simulink model "CM650A_HwTq0Meas"  (R2013b)
settings: Solver=FixedStepDiscrete  StartTime=0.0  StopTime=20  FixedStep=0.002  RelTol=1e-3
values from neighbouring files (symbols this model uses):
  ELECGLBPRM_HWTQOFFS_HWNWTMTR_F32 = DataDict.Constant    [CM650A_HwTq0Meas_DataDict.m]
  ELECGLBPRM_HWTQSATNLOWRLIM_HWNWTMTR_F32 = DataDict.Constant    [CM650A_HwTq0Meas_DataDict.m]
  ELECGLBPRM_HWTQSATNUPPRLIM_HWNWTMTR_F32 = DataDict.Constant    [CM650A_HwTq0Meas_DataDict.m]
  ELECGLBPRM_HWTQSCA_ULS_F32 = DataDict.Constant    [CM650A_HwTq0Meas_DataDict.m]
  ELECGLBPRM_NOFLT_CNT_U08 = DataDict.Constant    [CM650A_HwTq0Meas_DataDict.m]
  ELECGLBPRM_OFFSTRIMNOTPRFM_CNT_U08 = DataDict.Constant    [CM650A_HwTq0Meas_DataDict.m]
  ELECGLBPRM_PRTCLFLT_CNT_U08 = DataDict.Constant    [CM650A_HwTq0Meas_DataDict.m]
  ELECGLBPRM_SNSRINTFLT_CNT_U08 = DataDict.Constant    [CM650A_HwTq0Meas_DataDict.m]
  FLTINJ_HWTQ0MEAS_HWTQ0 = DataDict.Constant    [CM650A_HwTq0Meas_DataDict.m]
  FLTINJ_HWTQ0MEAS_TESTOK0 = DataDict.Constant    [CM650A_HwTq0Meas_DataDict.m]
  HwTq0MeasHwTq0PrtclFltFailStep = DataDict.Calibration    [CM650A_HwTq0Meas_DataDict.m]
  HwTq0MeasHwTq0PrtclFltPassStep = DataDict.Calibration    [CM650A_HwTq0Meas_DataDict.m]
  RACKLIMRCCWEOTSCA_ULS_F32 = DataDict.Constant    [CM650A_HwTq0Meas_DataDict.m]
  RACKLIMRCWEOTSCA_ULS_F32 = DataDict.Constant    [CM650A_HwTq0Meas_DataDict.m]
undefined symbols (not defined in the file or in its folder): NtcNr1, NtcSts1, sigbuilder_block, SigQlfr1
libraries: simulink x23, NxtrNvM x3, NxtrLim x2
(part 1 of 3)
settings Model: CovMetricSettings=dcmtrzoiw  CovFilter=CM650A_HwTq0Meas_covfilter  CovHTMLOptions=-sRT=1 -aTS=1 -bRG=1 -bTC=1 -hTR=0 -nFC=0 -scm=1 -bcm=1 -xEv=0  CovModelRefEnable=off  BufferReuse=off  Creator=CZ68DS  LastModifiedBy=FZG88Y
settings SolverCC: AutoInsertRateTranBlk=on
settings DataIOCC: SaveFormat=StructureWithTime
settings OptimizationCC: BlockReduction=off  DefaultUnderspecifiedDataType=single  OptimizeBlockIOStorage=off  BufferReuse=off  ExpressionFolding=off  LocalBlockOutputs=off  OptimizeModelRefInitCode=on  LifeSpan=1
settings DebuggingCC: MultiTaskDSMMsg=warning  FrameProcessingCompatibilityMsg=error
settings HardwareCC: ProdIntDivRoundTo=Zero  ProdEndianess=LittleEndian  ProdHWDeviceType=Generic->Custom  TargetIntDivRoundTo=Zero  TargetEndianess=LittleEndian  TargetHWDeviceType=Generic->Custom
settings RTWCC: SystemTargetFile=ert.tlc  TemplateMakefile=ert_default_tmf  Description=Embedded Coder  ProcessScript=ert_make_rtw_hook
settings CodeAppCC: IgnoreCustomStorageClasses=off
settings ERTTargetCC: CodeReplacementLibrary=C89/C90 (ANSI)  GenerateSampleERTMain=on  ERTCustomFileTemplate=example_file_process.tlc

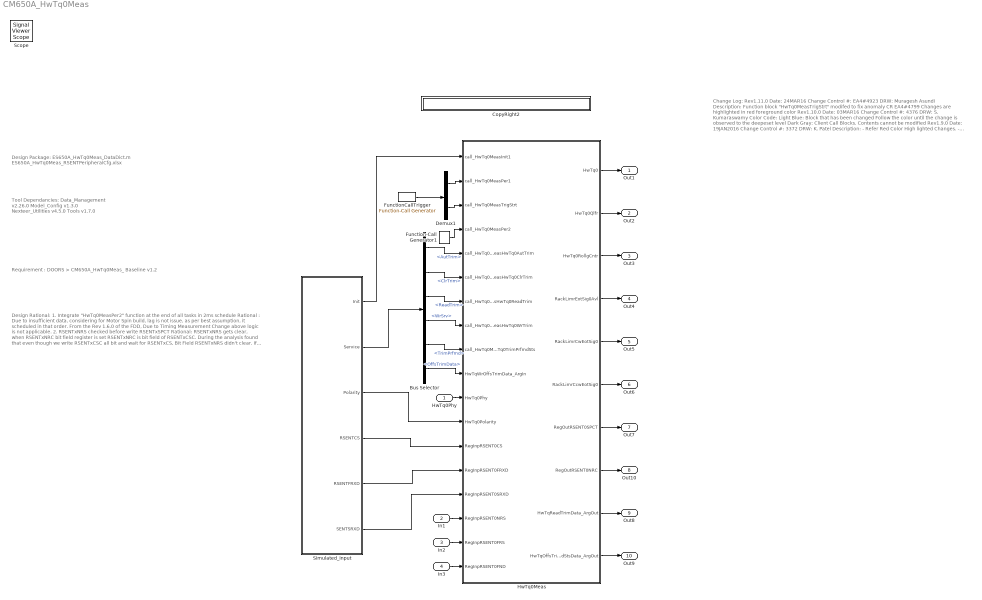
== system CM650A_HwTq0Meas ==
  note: Design Package:
      |
      | ES650A_HwTq0Meas_DataDict.m
      | ES650A_HwTq0Meas_RSENTPeripheralCfg.xlsx
  note: Change Log:
      |
      | Rev1.11.0
      | Date: 24MAR16
      | Change Control #: EA4#4923
      | DRW: Muragesh Asundi
      | Description:
      | Function block "HwTq0MeasTrigStrt" modifed to fix anomaly CR EA4#4799
      | Changes are highlighted in red foreground color
      |
      | Rev1.10.0
      | Date: 03MAR16
      | Change Control #: 4376
      | DRW: S. Kumaraswamy
      | Color Code:
      | Light Blue:	Block that has been changed
      | 				Follow the color until the change is observed to the deepeset level
      | Dark Gray:	Client Call Blocks. Contents cannot be modified
      |
      | Rev1.9.0
      | Date: 19JAN2016
      | Change Control #: 3372
      | DRW: K. Patel
      | Description:
      | - Refer Red Color High lighted Changes.
      | -  "CM650A_HwTq0Meas_RSENTPeripheralCfg.xlsx" change
      |
      | Rev1.8.0
      | Date: 16DEC2015
      | Change Control #: 3155
      | DRW: K. Patel
      | Description:
      | - Refer Red Color High lighted Changes.
      |
      | Rev1.7.0
      | Date: 22OCT2015
      | Change Control #: EA4#2221
      | DRW: K. Patel
      | Description:
      | - Slow Serial Message Fix
      | - EA4 Naming Correction for HwTq0MeasTrigStart
      |
      | Rev1.6.0
      | Date: 09OCT2015
      | Change Control #: EA4#1919
      | DRW: K. Patel
      | Description:
      | - Torque Trigger server function, Per3 change to Per2, Missing Message Counter add per1,
      | remove register from "CM650A_HwTq0Meas_RSENTPeripheralCfg.xlsx", change sync time to 16
      |
      | Rev1.5.0
      | Date: 02OCT2015
      | Change Control #: EA4#1811
      | DRW: Pallav G/Muragesh A (KPIT)
      | Description:
      | - Corrected output signal names RickLimrCcwEotSig0, RickLimrCwEotSig0 to RackLimrCcwEotSig0 and RackLimrCwEotSig0 respectively
      | - Range limiter added for above two output signals
      |
      | Rev1.4.0
      | Date: 20AUG2015
      | Change Control #: WCR-EA4#1283
      | DRW: K. Patel
      | Description:
      | - Rack Limiter End of Travel Signal 0 Data Read Function added
      |
      | Rev1.3.0
      | Date: 30JUL2015
      | Change Control #: WCR-EA4#1163, EA4#1222
      | DRW: K. Patel
      | Description:
      | - m file correction, Tick Time change from 1us to 1.2us
      | - Global Constant
      |
      | Rev1.2.0
      | Date: 29JUN2015
      | Change Control #: WCR-EA4#993
      | DRW: K. Patel
      | Description:
      | - Fault Injection added
      | - Trim Services Added
      | - Remove Mask in protocol evaluation & use field level register for input
      |
      | Rev1.1.0
      | Date: 30MAR2015
      | Change Control #: WCR-EA4#531
      | DRW: K. Patel
      | Description:
      | - Constant Added to m file and name corrected as per autosar
      | - Configuration Change in Init added
      |
      | Rev: 1.0.1
      | Date: 30MAR2015
      | Change Control #: WCR-EA4#425
      | DRW: K. Patel
      | Description:
      | - DebStep Cal range change and unit corrected in M file
      | - HwTq0Phy terminate out side of Init function as per Software Recommandation
      | - HwTq0MeasInit start with index 1 corrected as per EA4 meeting decision
      |
      | DRW: Keyur Patel
      | Description:
      | - Model intent to implement EA4 SENT0 based Digital Torque implementation for T1xx.
      |    model runs at three different function rate:
      |       1) Init - Configure Peripheral
      |       2) 2ms - Running SENT data, protocol fault, HwNm calculation, SENT trigger.
      |       3) 100ms - Per3 Trim Not Performed evaluation
      |       4) Event Trim Service - Auto, Clear, Write, Read, Trim Performed Status
      | - Fault Injection added
      | - Copyright Blocks added to each layer
      |
      | Rev: 100
      | Date: 6MAR2015
      | Change Control #: WCR-EA4#152
      | DRW: K. Patel
      | Description:
      | - Initial Release
  note: Tool Dependancies:
      |
      | Data_Management v2.26.0
      | Model_Config v1.3.0
      | Nexteer_Utilities v4.5.0
      | Tools v1.7.0
  note: Requirement :
      |
      | DOORS > CM650A_HwTq0Meas_ Baseline v1.2
  note: Design Rational:
      |
      | 1. Integrate "HwTq0MeasPer2" function at the end of all tasks in 2ms schedule
      | Rational : Due to insufficient data, considering for Motor Spin build, lag is not
      | issue, as per best assumption, it scheduled in that order.
      |
      | From the Rev 1.6.0 of the FDD, Due to Timing Measurement Change above
      | logic is not applicable.
      |
      | 2. RSENTxNRS checked before write RSENTxSPCT
      | Rational: RSENTxNRS gets clear, when RSENTxNRC bit field register is set
      | RSENTxNRC is bit field of RSENTxCSC. During the analysis found that
      | even though we write RSENTxCSC all bit and wait for RSENTxCS, Bit Field
      | RSENTxNRS didn't clear. If RSENTxNRS is set then writing RSENTxSPCT,
      | Peripheral will not output Pulse.
      |
      | Also found that RSENTxCS didn't clear itself, so need to always clear after
      | read message.
      |
      | 3. RSENTxSPCT need to write first to verify RSENTxNRS status
      | Rational : As per the Renesas User's hardware manual v1.0 -
      | Section 19 -SPC function, "Writing to RSENTnSPCT.TLL requests a
      | SPC trigger transmission. After writing to RSENTnSPCT.TLL, the CPU
      | should read RSENTnCS.NRS to check whether the previous request was
      | completed or not."
  HwTq0Phy : Inport
  In1 : Inport  Port=2
  In2 : Inport  Port=3
  In3 : Inport  Port=4
  Bus Selector : BusSelector  OutputSignals=AutTrim,ClrTrim,ReadTrim,WrSrv,TrimPrfmd,OffsTrimData
  CopyRight2 : Subsystem  Description=|  mask(Copyright Information){none=on}
      | Copyright info block.                                               
      |                                                                     
      | Place copyright information at the top of every subsystem in design.
      mask prompts: none "No parameters"
      mask help: Place copyright information at the top of every subsystem in design.
      mask Display:
      | NxtrConf = 'Nexteer Confidential';
      | 
      | sys = bdroot; %handle for the current model ("system")
      | first = get_param(sys,'Created');
      | first = first(end-3:end);  %year is last four digits
      | 
      | last = get_param(sys,'LastModifiedDate');
      | if isempty(last)
      |     last = datestr(now,'yyyy');
      | else
      |     last = last(end-3:end);
      | end
      | 
      | if strcmp(first,last)
      |     fprintf('%s -- Copyright %s Nexteer',NxtrConf,first)
      | else
      |     fprintf('%s -- %s%s- %s Nexteer',NxtrConf,char(169),first,last)
      | end
  Demux1 : Demux  Outputs=2
  Function-Call Generator1 : simulink/Ports & Subsystems/Function-Call Generator  sample_time=0.100  numberOfIterations=1
  FunctionCallTrigger : simulink/Ports & Subsystems/Function-Call Generator  RequirementInfo={} %GIDa_461051ca_e299_4da2_91c0_e73e41056377  sample_time=0.002  numberOfIterations=1
  HwTq0Meas : Subsystem  Priority=1
      settings: AttributesFormatString=Priority = %<Priority>
  Simulated_Input : Subsystem  Description=Do not Code this block
      settings: AttributesFormatString=%<Description>
  Out1 : Outport
  Out2 : Outport  Port=2
  Out3 : Outport  Port=3
  Out4 : Outport  Port=4
  Out5 : Outport  Port=5
  Out6 : Outport  Port=6
  Out7 : Outport  Port=7
  Out10 : Outport  Port=8
  Out8 : Outport  Port=9
  Out9 : Outport  Port=10
  Scope : SignalViewerScope  IOType=viewer  SampleTime=-1  RefreshTime=0.035000
      settings: YMin=-10  YMax=10
  wires:
  FunctionCallTrigger/1 -> Demux1/1
  HwTq0Phy/1 -> HwTq0Meas/11(HwTq0Phy)
  Simulated_Input/3(Polarity) -> HwTq0Meas/12(HwTq0Polarity)
  HwTq0Meas/3(HwTq0RollgCntr) -> Out3/1
  HwTq0Meas/1(HwTq0) -> Out1/1
  HwTq0Meas/2(HwTq0Qlfr) -> Out2/1
  HwTq0Meas/7(RegOutRSENT0SPCT) -> Out7/1
  Function-Call Generator1/1 -> HwTq0Meas/4(call_HwTq0MeasPer2)
  Demux1/1 -> HwTq0Meas/2(call_HwTq0MeasPer1)
  Demux1/2 -> HwTq0Meas/3(call_HwTq0MeasTrigStrt)
  Bus Selector/1 -> HwTq0Meas/5(call_HwTq0MeasHwTq0AutTrim)  "<AutTrim>"
  Bus Selector/2 -> HwTq0Meas/6(call_HwTq0MeasHwTq0ClrTrim)  "<ClrTrim>"
  Bus Selector/3 -> HwTq0Meas/7(call_HwTq0MeasHwTq0ReadTrim)  "<ReadTrim>"
  Bus Selector/4 -> HwTq0Meas/8(call_HwTq0MeasHwTq0WrTrim)  "<WrSrv>"
  Bus Selector/5 -> HwTq0Meas/9(call_HwTq0MeasHwTq0TrimPrfmdSts)  "<TrimPrfmd>"
  Bus Selector/6 -> HwTq0Meas/10(HwTqWrOffsTrimData_ArgIn)  "<OffsTrimData>"
  Simulated_Input/1(Init) -> HwTq0Meas/1(call_HwTq0MeasInit1)
  Simulated_Input/2(Service) -> Bus Selector/1
  Simulated_Input/4(RSENTCS) -> HwTq0Meas/13(RegInpRSENT0CS)
  Simulated_Input/5(RSENTFRXD) -> HwTq0Meas/14(RegInpRSENT0FRXD)
  HwTq0Meas/9(HwTqReadTrimData_ArgOut) -> Out8/1
  HwTq0Meas/10(HwTqOffsTrimPrfmdStsData_ArgOut) -> Out9/1
  HwTq0Meas/4(RackLimrEotSig0Avl) -> Out4/1
  HwTq0Meas/5(RackLimrCwEotSig0) -> Out5/1
  HwTq0Meas/6(RackLimrCcwEotSig0) -> Out6/1
  Simulated_Input/6(SENTSRXD) -> HwTq0Meas/15(RegInpRSENT0SRXD)
  HwTq0Meas/8(RegOutRSENT0NRC) -> Out10/1
  In1/1 -> HwTq0Meas/16(RegInpRSENT0NRS)
  In2/1 -> HwTq0Meas/17(RegInpRSENT0FRS)
  In3/1 -> HwTq0Meas/18(RegInpRSENT0FND)

== system CM650A_HwTq0Meas/CopyRight2 ==

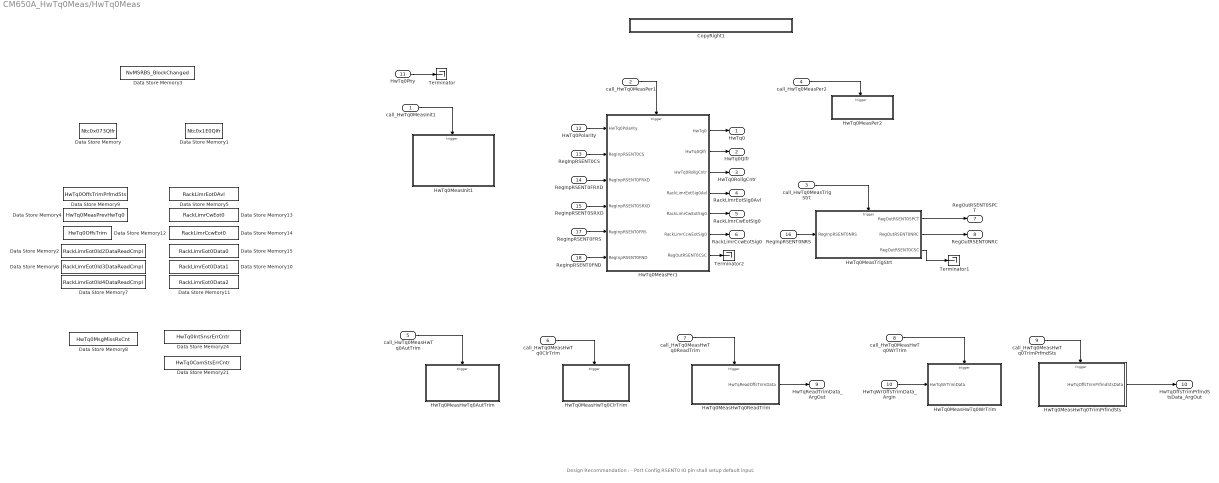
== system CM650A_HwTq0Meas/HwTq0Meas ==
  note: Design Recommandation :
      |
      | - Port Config RSENT0 IO pin shall setup default input.
  call_HwTq0MeasInit1 : Inport
  call_HwTq0MeasPer1 : Inport  Description=2ms  Port=2
      settings: AttributesFormatString=%<Description>
  call_HwTq0MeasTrigStrt : Inport  Description=Event  Port=3
      settings: AttributesFormatString=%<Description>
  call_HwTq0MeasPer2 : Inport  Description=100ms  Port=4
      settings: AttributesFormatString=%<Description>
  call_HwTq0MeasHwTq0AutTrim : Inport  Description=Event  Port=5
      settings: AttributesFormatString=%<Description>
  call_HwTq0MeasHwTq0ClrTrim : Inport  Description=Event  Port=6
      settings: AttributesFormatString=%<Description>
  call_HwTq0MeasHwTq0ReadTrim : Inport  Description=Event  Port=7
      settings: AttributesFormatString=%<Description>
  call_HwTq0MeasHwTq0WrTrim : Inport  Description=Event  Port=8
      settings: AttributesFormatString=%<Description>
  call_HwTq0MeasHwTq0TrimPrfmdSts : Inport  Description=Event  Port=9
      settings: AttributesFormatString=%<Description>
  HwTqWrOffsTrimData_ArgIn : Inport  Port=10
  HwTq0Phy : Inport  Port=11
  HwTq0Polarity : Inport  Port=12  OutDataTypeStr=int8
  RegInpRSENT0CS : Inport  Port=13
  RegInpRSENT0FRXD : Inport  Port=14
  RegInpRSENT0SRXD : Inport  Port=15
  RegInpRSENT0NRS : Inport  Port=16
  RegInpRSENT0FRS : Inport  Port=17
  RegInpRSENT0FND : Inport  Port=18
  CopyRight1 : Subsystem  Description=|  mask(Copyright Information){none=on}
      | Copyright info block.                                               
      |                                                                     
      | Place copyright information at the top of every subsystem in design.
      mask prompts: none "No parameters"
      mask help: Place copyright information at the top of every subsystem in design.
      mask Display:
      | NxtrConf = 'Nexteer Confidential';
      | 
      | sys = bdroot; %handle for the current model ("system")
      | first = get_param(sys,'Created');
      | first = first(end-3:end);  %year is last four digits
      | 
      | last = get_param(sys,'LastModifiedDate');
      | if isempty(last)
      |     last = datestr(now,'yyyy');
      | else
      |     last = last(end-3:end);
      | end
      | 
      | if strcmp(first,last)
      |     fprintf('%s -- Copyright %s Nexteer',NxtrConf,first)
      | else
      |     fprintf('%s -- %s%s- %s Nexteer',NxtrConf,char(169),first,last)
      | end
  Data Store Memory10 : DataStoreMemory  DataStoreName=RackLimrEot0Data1  ReadBeforeWriteMsg=warning  WriteAfterWriteMsg=warning  WriteAfterReadMsg=warning  StateMustResolveToSignalObject=on
  Data Store Memory11 : DataStoreMemory  DataStoreName=RackLimrEot0Data2  ReadBeforeWriteMsg=warning  WriteAfterWriteMsg=warning  WriteAfterReadMsg=warning  StateMustResolveToSignalObject=on
  Data Store Memory12 : DataStoreMemory  DataStoreName=HwTq0OffsTrim  ReadBeforeWriteMsg=warning  WriteAfterWriteMsg=warning  WriteAfterReadMsg=warning
  Data Store Memory13 : DataStoreMemory  DataStoreName=RackLimrCwEot0  ReadBeforeWriteMsg=warning  WriteAfterWriteMsg=warning  WriteAfterReadMsg=warning  StateMustResolveToSignalObject=on
  Data Store Memory14 : DataStoreMemory  DataStoreName=RackLimrCcwEot0  ReadBeforeWriteMsg=warning  WriteAfterWriteMsg=warning  WriteAfterReadMsg=warning  StateMustResolveToSignalObject=on
  Data Store Memory15 : DataStoreMemory  DataStoreName=RackLimrEot0Data0  ReadBeforeWriteMsg=warning  WriteAfterWriteMsg=warning  WriteAfterReadMsg=warning  StateMustResolveToSignalObject=on
  Data Store Memory2 : DataStoreMemory  DataStoreName=RackLimrEot0Id2DataReadCmpl  ReadBeforeWriteMsg=warning  WriteAfterWriteMsg=warning  WriteAfterReadMsg=warning  StateMustResolveToSignalObject=on
  Data Store Memory21 : DataStoreMemory  DataStoreName=HwTq0ComStsErrCntr  ReadBeforeWriteMsg=warning  WriteAfterWriteMsg=warning  WriteAfterReadMsg=warning  StateMustResolveToSignalObject=on
  Data Store Memory24 : DataStoreMemory  DataStoreName=HwTq0IntSnsrErrCntr  ReadBeforeWriteMsg=warning  WriteAfterWriteMsg=warning  WriteAfterReadMsg=warning  StateMustResolveToSignalObject=on
  Data Store Memory4 : DataStoreMemory  DataStoreName=HwTq0MeasPrevHwTq0  ReadBeforeWriteMsg=warning  WriteAfterWriteMsg=warning  WriteAfterReadMsg=warning
  Data Store Memory5 : DataStoreMemory  DataStoreName=RackLimrEot0Avl  ReadBeforeWriteMsg=warning  WriteAfterWriteMsg=warning  WriteAfterReadMsg=warning  StateMustResolveToSignalObject=on
  Data Store Memory6 : DataStoreMemory  DataStoreName=RackLimrEot0Id3DataReadCmpl  ReadBeforeWriteMsg=warning  WriteAfterWriteMsg=warning  WriteAfterReadMsg=warning  StateMustResolveToSignalObject=on
  Data Store Memory7 : DataStoreMemory  DataStoreName=RackLimrEot0Id4DataReadCmpl  ReadBeforeWriteMsg=warning  WriteAfterWriteMsg=warning  WriteAfterReadMsg=warning  StateMustResolveToSignalObject=on
  Data Store Memory8 : DataStoreMemory  DataStoreName=HwTq0MsgMissRxCnt  ReadBeforeWriteMsg=warning  WriteAfterWriteMsg=warning  WriteAfterReadMsg=warning  StateMustResolveToSignalObject=on
  Data Store Memory9 : DataStoreMemory  DataStoreName=HwTq0OffsTrimPrfmdSts  ReadBeforeWriteMsg=warning  WriteAfterWriteMsg=warning  WriteAfterReadMsg=warning
  Data Store Memory : DataStoreMemory  DataStoreName=Ntc0x073Qlfr  ReadBeforeWriteMsg=warning  WriteAfterWriteMsg=warning  WriteAfterReadMsg=warning  OutDataTypeStr=uint8
      settings: AttributesFormatString=|
      | Simulation Purpose Only.
      | Do Not Code this block
      | Diagnostic Manager Owns this requirement
  Data Store Memory1 : DataStoreMemory  DataStoreName=Ntc0x1E0Qlfr  ReadBeforeWriteMsg=warning  WriteAfterWriteMsg=warning  WriteAfterReadMsg=warning  OutDataTypeStr=uint8
      settings: AttributesFormatString=|
      | Simulation Purpose Only.
      | Do Not Code this block
      | Diagnostic Manager Owns this requirement
  Data Store Memory3 : DataStoreMemory  DataStoreName=NvMSRBS_BlockChanged  ReadBeforeWriteMsg=warning  WriteAfterWriteMsg=warning  WriteAfterReadMsg=warning  OutDataTypeStr=uint8
      settings: AttributesFormatString=|
      | Simulation Purpose Only.
      | Do Not Code this block
      | Diagnostic Manager Owns this requirement
  HwTq0MeasHwTq0AutTrim : Subsystem  RequirementInfo={'linktype_rmi_doors' '0000c468 (/ESG Group/FDD Module Requirements/EA4 Specific/CM650A_HwTq0Meas)' '#CM650A_56' 'true' 'REQ: CM650A_56' '' } %GIDa_78a0150d_b2b2_4893_8cf0_7a267cd87682  Priority=10  TreatAsAtomicUnit=on
      settings: AttributesFormatString=Priority=%<Priority>
  HwTq0MeasHwTq0ClrTrim : Subsystem  RequirementInfo={'linktype_rmi_doors' '0000c468 (/ESG Group/FDD Module Requirements/EA4 Specific/CM650A_HwTq0Meas)' '#CM650A_54' 'true' 'REQ: CM650A_54' '' } %GIDa_9d8bf3ad_e540_4a5e_ad4c_eb940ac157ad  Priority=10  TreatAsAtomicUnit=on
      settings: AttributesFormatString=Priority=%<Priority>
  HwTq0MeasHwTq0ReadTrim : Subsystem  RequirementInfo={'linktype_rmi_doors' '0000c468 (/ESG Group/FDD Module Requirements/EA4 Specific/CM650A_HwTq0Meas)' '#CM650A_52' 'true' 'REQ: CM650A_52' '' } %GIDa_4c78535b_9e38_436f_a670_46438fd62cfe  Priority=10  TreatAsAtomicUnit=on
      settings: AttributesFormatString=Priority=%<Priority>
  HwTq0MeasHwTq0TrimPrfmdSts : Subsystem  RequirementInfo={'linktype_rmi_doors' '0000c468 (/ESG Group/FDD Module Requirements/EA4 Specific/CM650A_HwTq0Meas)' '#CM650A_53' 'true' 'REQ: CM650A_53' '' } %GIDa_05e70ef2_f8d5_471c_a4a3_b95d94c92180  Priority=10  TreatAsAtomicUnit=on
      settings: AttributesFormatString=Priority=%<Priority>
  HwTq0MeasHwTq0WrTrim : Subsystem  RequirementInfo={'linktype_rmi_doors' '0000c468 (/ESG Group/FDD Module Requirements/EA4 Specific/CM650A_HwTq0Meas)' '#CM650A_55' 'true' 'REQ: CM650A_55' '' } %GIDa_58f23a20_9e17_4252_b727_77362ca5c7be  Priority=10  TreatAsAtomicUnit=on
      settings: AttributesFormatString=Priority=%<Priority>
  HwTq0MeasInit1 : Subsystem  TreatAsAtomicUnit=on
  HwTq0MeasPer1 : Subsystem  RequirementInfo={'linktype_rmi_doors' '0000c468 (/ESG Group/FDD Module Requirements/EA4 Specific/CM650A_HwTq0Meas)' '#CM650A_22' 'true' 'REQ: CM650A_22' '' ; 'linktype_rmi_doors' '0000c468 (/ESG Group/FDD Module Requirements/EA4 Specific/CM650A_HwTq0Meas)' '#CM650A_38' 'true' 'REQ: CM650A_38' '' } %GIDa_31b3da74_5937_4fb2_b915_5c5c5e5711e7  TreatAsAtomicUnit=on
  HwTq0MeasPer2 : Subsystem  RequirementInfo={'linktype_rmi_doors' '0000c468 (/ESG Group/FDD Module Requirements/EA4 Specific/CM650A_HwTq0Meas)' '#CM650A_63' 'true' 'REQ: CM650A_63' '' } %GIDa_c89b04b6_b4c1_41bf_b3f8_efad30b9fb82  Priority=8  TreatAsAtomicUnit=on
      settings: AttributesFormatString=Priority=%<Priority>
  HwTq0MeasTrigStrt : Subsystem  RequirementInfo={'linktype_rmi_doors' '0000c468 (/ESG Group/FDD Module Requirements/EA4 Specific/CM650A_HwTq0Meas)' '#CM650A_50' 'true' 'REQ: CM650A_50' '' } %GIDa_ac2e4248_233e_47e7_8dc6_e55969fb5c4e  TreatAsAtomicUnit=on
  Terminator : Terminator
  Terminator1 : Terminator
  Terminator2 : Terminator
  HwTq0 : Outport
  HwTq0Qlfr : Outport  Port=2
  HwTq0RollgCntr : Outport  Port=3
  RackLimrEotSig0Avl : Outport  Port=4
  RackLimrCwEotSig0 : Outport  Port=5
  RackLimrCcwEotSig0 : Outport  Port=6
  RegOutRSENT0SPCT : Outport  Port=7
  RegOutRSENT0NRC : Outport  Port=8
  HwTqReadTrimData_ArgOut : Outport  Port=9
  HwTqOffsTrimPrfmdStsData_ArgOut : Outport  Port=10
  wires:
  call_HwTq0MeasPer1/1 -> HwTq0MeasPer1/Trigger
  call_HwTq0MeasInit1/1 -> HwTq0MeasInit1/Trigger
  HwTq0MeasPer1/1(HwTq0) -> HwTq0/1
  HwTq0MeasPer1/2(HwTq0Qlfr) -> HwTq0Qlfr/1
  HwTq0MeasPer1/3(HwTq0RollgCntr) -> HwTq0RollgCntr/1
  call_HwTq0MeasTrigStrt/1 -> HwTq0MeasTrigStrt/Trigger
  HwTq0Polarity/1 -> HwTq0MeasPer1/1(HwTq0Polarity)
  HwTq0MeasTrigStrt/1(RegOutRSENT0SPCT) -> RegOutRSENT0SPCT/1
  HwTq0Phy/1 -> Terminator/1
  call_HwTq0MeasHwTq0AutTrim/1 -> HwTq0MeasHwTq0AutTrim/Trigger
  call_HwTq0MeasHwTq0ClrTrim/1 -> HwTq0MeasHwTq0ClrTrim/Trigger
  call_HwTq0MeasHwTq0ReadTrim/1 -> HwTq0MeasHwTq0ReadTrim/Trigger
  call_HwTq0MeasHwTq0WrTrim/1 -> HwTq0MeasHwTq0WrTrim/Trigger
  call_HwTq0MeasHwTq0TrimPrfmdSts/1 -> HwTq0MeasHwTq0TrimPrfmdSts/Trigger
  HwTqWrOffsTrimData_ArgIn/1 -> HwTq0MeasHwTq0WrTrim/1(HwTqWrTrimData)
  HwTq0MeasHwTq0ReadTrim/1(HwTqReadOffsTrimData) -> HwTqReadTrimData_ArgOut/1
  HwTq0MeasHwTq0TrimPrfmdSts/1(HwTqOffsTrimPrfmdStsData) -> HwTqOffsTrimPrfmdStsData_ArgOut/1
  call_HwTq0MeasPer2/1 -> HwTq0MeasPer2/Trigger
  RegInpRSENT0CS/1 -> HwTq0MeasPer1/2(RegInpRSENT0CS)
  RegInpRSENT0FRXD/1 -> HwTq0MeasPer1/3(RegInpRSENT0FRXD)
  RegInpRSENT0SRXD/1 -> HwTq0MeasPer1/4(RegInpRSENT0SRXD)
  HwTq0MeasPer1/4(RackLimrEotSig0Avl) -> RackLimrEotSig0Avl/1
  HwTq0MeasPer1/5(RackLimrCwEotSig0) -> RackLimrCwEotSig0/1
  HwTq0MeasPer1/6(RackLimrCcwEotSig0) -> RackLimrCcwEotSig0/1
  HwTq0MeasTrigStrt/2(RegOutRSENT0NRC) -> RegOutRSENT0NRC/1
  HwTq0MeasTrigStrt/3(RegOutRSENT0CSC) -> Terminator1/1
  HwTq0MeasPer1/7(RegOutRSENT0CSC) -> Terminator2/1
  RegInpRSENT0FRS/1 -> HwTq0MeasPer1/5(RegInpRSENT0FRS)
  RegInpRSENT0FND/1 -> HwTq0MeasPer1/6(RegInpRSENT0FND)
  RegInpRSENT0NRS/1 -> HwTq0MeasTrigStrt/1(RegInpRSENT0NRS)

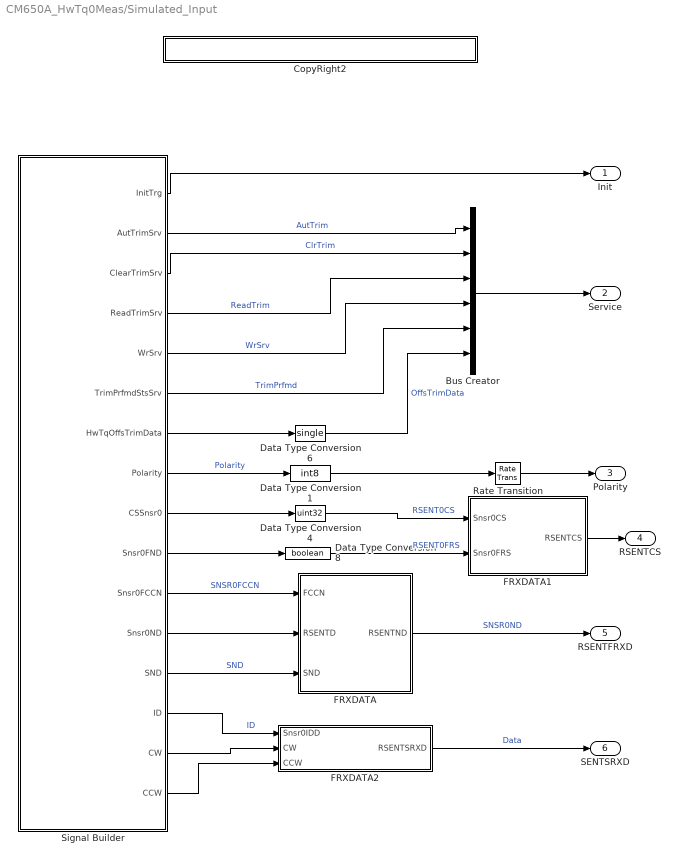
== system CM650A_HwTq0Meas/Simulated_Input ==
  Bus Creator : BusCreator  Inputs=6
  CopyRight2 : Subsystem  Description=|  mask(Copyright Information){none=on}
      | Copyright info block.                                               
      |                                                                     
      | Place copyright information at the top of every subsystem in design.
      mask prompts: none "No parameters"
      mask help: Place copyright information at the top of every subsystem in design.
      mask Display:
      | NxtrConf = 'Nexteer Confidential';
      | 
      | sys = bdroot; %handle for the current model ("system")
      | first = get_param(sys,'Created');
      | first = first(end-3:end);  %year is last four digits
      | 
      | last = get_param(sys,'LastModifiedDate');
      | if isempty(last)
      |     last = datestr(now,'yyyy');
      | else
      |     last = last(end-3:end);
      | end
      | 
      | if strcmp(first,last)
      |     fprintf('%s -- Copyright %s Nexteer',NxtrConf,first)
      | else
      |     fprintf('%s -- %s%s- %s Nexteer',NxtrConf,char(169),first,last)
      | end
  Data Type Conversion1 : DataTypeConversion  OutDataTypeStr=int8
  Data Type Conversion4 : DataTypeConversion  OutDataTypeStr=uint32
  Data Type Conversion6 : DataTypeConversion  OutDataTypeStr=single
  Data Type Conversion8 : DataTypeConversion  OutDataTypeStr=boolean
  FRXDATA : Subsystem
  FRXDATA1 : Subsystem
  FRXDATA2 : Subsystem
  Rate Transition : RateTransition
  Signal Builder : Subsystem  Tag=STV Subsys  LoadFcn=sigbuilder_block('load');  StartFcn=sigbuilder_block('start');  StopFcn=sigbuilder_block('stop');  ClipboardFcn=sigbuilder_block('clipboard');  mask(Sigbuilder block){}
      mask help: Simulink:masks:SigbuilderBlock_MD
      mask init:
      | if ~strcmp(get_param(bdroot(gcbh),'SimulationStatus'),'stopped') tuvar = sigbuilder_block('maskInit'); end
      settings: CopyFcn=sigbuilder_block('copy');  DeleteFcn=sigbuilder_block('delete');  ModelCloseFcn=sigbuilder_block('modelClose');  PreSaveFcn=sigbuilder_block('preSave');  PauseFcn=sigbuilder_block('pause');  ContinueFcn=sigbuilder_block('continue');  NameChangeFcn=sigbuilder_block('namechange');  OpenFcn=sigbuilder_block('open',[57 0 967.5 519 ]);  CloseFcn=sigbuilder_block('close');
      mask Display: plot(0, 0, 100, 100,[2, 2, 32, 32, 2], [68, 8, 8, 68, 68],[32, 2], [38, 38], [32, 19, 2],[53, 60, 44], [32, 17, 17, 2],[16, 16, 31, 31]);txt = getActiveGroup(gcbh);text(2, 100, txt,'verticalAlignment', 'top');
  Init : Outport
  Service : Outport  Port=2
  Polarity : Outport  Port=3
  RSENTCS : Outport  Port=4
  RSENTFRXD : Outport  Port=5
  SENTSRXD : Outport  Port=6
  wires:
  Data Type Conversion6/1 -> Bus Creator/6  "OffsTrimData"
  Signal Builder/11(Snsr0FCCN) -> FRXDATA/1(FCCN)  "SNSR0FCCN"
  Data Type Conversion8/1 -> FRXDATA1/2(Snsr0FRS)  "RSENT0FRS"
  Data Type Conversion4/1 -> FRXDATA1/1(Snsr0CS)  "RSENT0CS"
  Rate Transition/1 -> Polarity/1
  Data Type Conversion1/1 -> Rate Transition/1
  FRXDATA/1(RSENTND) -> RSENTFRXD/1  "SNSR0ND"
  Bus Creator/1 -> Service/1
  Signal Builder/10(Snsr0FND) -> Data Type Conversion8/1
  Signal Builder/9(CSSnsr0) -> Data Type Conversion4/1
  Signal Builder/12(Snsr0ND) -> FRXDATA/2(RSENTD)
  Signal Builder/2(AutTrimSrv) -> Bus Creator/1  "AutTrim"
  Signal Builder/3(ClearTrimSrv) -> Bus Creator/2  "ClrTrim"
  Signal Builder/4(ReadTrimSrv) -> Bus Creator/3  "ReadTrim"
  Signal Builder/5(WrSrv) -> Bus Creator/4  "WrSrv"
  Signal Builder/6(TrimPrfmdStsSrv) -> Bus Creator/5  "TrimPrfmd"
  Signal Builder/7(HwTqOffsTrimData) -> Data Type Conversion6/1
  Signal Builder/1(InitTrg) -> Init/1
  Signal Builder/8(Polarity) -> Data Type Conversion1/1  "Polarity"
  Signal Builder/13(SND) -> FRXDATA/3(SND)  "SND"
  FRXDATA2/1(RSENTSRXD) -> SENTSRXD/1  "Data"
  Signal Builder/14(ID) -> FRXDATA2/1(Snsr0IDD)  "ID"
  Signal Builder/15(CW) -> FRXDATA2/2(CW)
  Signal Builder/16(CCW) -> FRXDATA2/3(CCW)
  FRXDATA1/1(RSENTCS) -> RSENTCS/1

== system CM650A_HwTq0Meas/HwTq0Meas/CopyRight1 ==

== system CM650A_HwTq0Meas/HwTq0Meas/HwTq0MeasHwTq0AutTrim ==
  function : TriggerPort
  CopyRight2 : Subsystem  Description=|  mask(Copyright Information){none=on}
      | Copyright info block.                                               
      |                                                                     
      | Place copyright information at the top of every subsystem in design.
      mask prompts: none "No parameters"
      mask help: Place copyright information at the top of every subsystem in design.
      mask Display:
      | NxtrConf = 'Nexteer Confidential';
      | 
      | sys = bdroot; %handle for the current model ("system")
      | first = get_param(sys,'Created');
      | first = first(end-3:end);  %year is last four digits
      | 
      | last = get_param(sys,'LastModifiedDate');
      | if isempty(last)
      |     last = datestr(now,'yyyy');
      | else
      |     last = last(end-3:end);
      | end
      | 
      | if strcmp(first,last)
      |     fprintf('%s -- Copyright %s Nexteer',NxtrConf,first)
      | else
      |     fprintf('%s -- %s%s- %s Nexteer',NxtrConf,char(169),first,last)
      | end
  NVM Shadow RAM : DataStoreWrite  RequirementInfo={} %GIDa_691c2588_2b45_48b9_9733_fd18f25444bb  DataStoreName=HwTq0OffsTrim
  NVM1 Shadow RAM : DataStoreWrite  RequirementInfo={'linktype_rmi_doors' '0000c468 (/ESG Group/FDD Module Requirements/EA4 Specific/CM650A_HwTq0Meas)' '#CM650A_49' 'true' 'REQ: CM650A_49' '' } %GIDa_8dfe2b68_c9bd_4b5f_9a85_4945a725dea6  DataStoreName=HwTq0OffsTrimPrfmdSts
  PIM : DataStoreRead  RequirementInfo={'linktype_rmi_doors' '0000c468 (/ESG Group/FDD Module Requirements/EA4 Specific/CM650A_HwTq0Meas)' '#CM650A_51' 'true' 'REQ: CM650A_51' '' } %GIDa_7720d852_cab6_4ee8_822b_ee5ddb596286  Priority=10  DataStoreName=HwTq0MeasPrevHwTq0
      settings: AttributesFormatString=Priority=%<Priority>
  Set : Constant
  Set Ram Block Status : NxtrNvM/Set Ram Block Status  FuncName=Set Ram Block Status  NvMBlockName=HwTq0Offs  VoidFuncRtn=on  BlockChanged_DSN=NvMSRBS_BlockChanged  Return_DSN=NvMSRBS_Return
      settings: AttributesFormatString=%<FuncName>
  Set3 : Constant  OutDataTypeStr=uint8
  wires:
  PIM/1 -> NVM Shadow RAM/1
  Set/1 -> NVM1 Shadow RAM/1
  Set3/1 -> Set Ram Block Status/1

== system CM650A_HwTq0Meas/HwTq0Meas/HwTq0MeasHwTq0ClrTrim ==
  function : TriggerPort
  Clear1 : Constant  Value=0  OutDataTypeStr=single
  Clear2 : Constant  Value=0
  CopyRight2 : Subsystem  Description=|  mask(Copyright Information){none=on}
      | Copyright info block.                                               
      |                                                                     
      | Place copyright information at the top of every subsystem in design.
      mask prompts: none "No parameters"
      mask help: Place copyright information at the top of every subsystem in design.
      mask Display:
      | NxtrConf = 'Nexteer Confidential';
      | 
      | sys = bdroot; %handle for the current model ("system")
      | first = get_param(sys,'Created');
      | first = first(end-3:end);  %year is last four digits
      | 
      | last = get_param(sys,'LastModifiedDate');
      | if isempty(last)
      |     last = datestr(now,'yyyy');
      | else
      |     last = last(end-3:end);
      | end
      | 
      | if strcmp(first,last)
      |     fprintf('%s -- Copyright %s Nexteer',NxtrConf,first)
      | else
      |     fprintf('%s -- %s%s- %s Nexteer',NxtrConf,char(169),first,last)
      | end
  NVM Shadow RAM : DataStoreWrite  RequirementInfo={} %GIDa_c01938bd_873a_4f20_8aad_b7368db2e426  DataStoreName=HwTq0OffsTrim
  NVM1 Shadow RAM : DataStoreWrite  RequirementInfo={'linktype_rmi_doors' '0000c468 (/ESG Group/FDD Module Requirements/EA4 Specific/CM650A_HwTq0Meas)' '#CM650A_49' 'true' 'REQ: CM650A_49' '' } %GIDa_7e661117_be14_43c5_b4c7_51bd14c3b186  DataStoreName=HwTq0OffsTrimPrfmdSts
  Set Ram Block Status : NxtrNvM/Set Ram Block Status  FuncName=Set Ram Block Status  NvMBlockName=HwTq0Offs  VoidFuncRtn=on  BlockChanged_DSN=NvMSRBS_BlockChanged  Return_DSN=NvMSRBS_Return
      settings: AttributesFormatString=%<FuncName>
  Set3 : Constant  OutDataTypeStr=uint8
  wires:
  Clear1/1 -> NVM Shadow RAM/1
  Clear2/1 -> NVM1 Shadow RAM/1
  Set3/1 -> Set Ram Block Status/1

== system CM650A_HwTq0Meas/HwTq0Meas/HwTq0MeasHwTq0ReadTrim ==
  function : TriggerPort
  CopyRight2 : Subsystem  Description=|  mask(Copyright Information){none=on}
      | Copyright info block.                                               
      |                                                                     
      | Place copyright information at the top of every subsystem in design.
      mask prompts: none "No parameters"
      mask help: Place copyright information at the top of every subsystem in design.
      mask Display:
      | NxtrConf = 'Nexteer Confidential';
      | 
      | sys = bdroot; %handle for the current model ("system")
      | first = get_param(sys,'Created');
      | first = first(end-3:end);  %year is last four digits
      | 
      | last = get_param(sys,'LastModifiedDate');
      | if isempty(last)
      |     last = datestr(now,'yyyy');
      | else
      |     last = last(end-3:end);
      | end
      | 
      | if strcmp(first,last)
      |     fprintf('%s -- Copyright %s Nexteer',NxtrConf,first)
      | else
      |     fprintf('%s -- %s%s- %s Nexteer',NxtrConf,char(169),first,last)
      | end
  NVM Shadow RAM : DataStoreRead  DataStoreName=HwTq0OffsTrim
  HwTqReadOffsTrimData : Outport
  wires:
  NVM Shadow RAM/1 -> HwTqReadOffsTrimData/1

== system CM650A_HwTq0Meas/HwTq0Meas/HwTq0MeasHwTq0TrimPrfmdSts ==
  function : TriggerPort
  CopyRight2 : Subsystem  Description=|  mask(Copyright Information){none=on}
      | Copyright info block.                                               
      |                                                                     
      | Place copyright information at the top of every subsystem in design.
      mask prompts: none "No parameters"
      mask help: Place copyright information at the top of every subsystem in design.
      mask Display:
      | NxtrConf = 'Nexteer Confidential';
      | 
      | sys = bdroot; %handle for the current model ("system")
      | first = get_param(sys,'Created');
      | first = first(end-3:end);  %year is last four digits
      | 
      | last = get_param(sys,'LastModifiedDate');
      | if isempty(last)
      |     last = datestr(now,'yyyy');
      | else
      |     last = last(end-3:end);
      | end
      | 
      | if strcmp(first,last)
      |     fprintf('%s -- Copyright %s Nexteer',NxtrConf,first)
      | else
      |     fprintf('%s -- %s%s- %s Nexteer',NxtrConf,char(169),first,last)
      | end
  Data Store Read1 : DataStoreRead  DataStoreName=HwTq0OffsTrimPrfmdSts
  HwTqOffsTrimPrfmdStsData : Outport
  wires:
  Data Store Read1/1 -> HwTqOffsTrimPrfmdStsData/1

== system CM650A_HwTq0Meas/HwTq0Meas/HwTq0MeasHwTq0WrTrim ==
  HwTqWrTrimData : Inport
  function : TriggerPort
  CopyRight2 : Subsystem  Description=|  mask(Copyright Information){none=on}
      | Copyright info block.                                               
      |                                                                     
      | Place copyright information at the top of every subsystem in design.
      mask prompts: none "No parameters"
      mask help: Place copyright information at the top of every subsystem in design.
      mask Display:
      | NxtrConf = 'Nexteer Confidential';
      | 
      | sys = bdroot; %handle for the current model ("system")
      | first = get_param(sys,'Created');
      | first = first(end-3:end);  %year is last four digits
      | 
      | last = get_param(sys,'LastModifiedDate');
      | if isempty(last)
      |     last = datestr(now,'yyyy');
      | else
      |     last = last(end-3:end);
      | end
      | 
      | if strcmp(first,last)
      |     fprintf('%s -- Copyright %s Nexteer',NxtrConf,first)
      | else
      |     fprintf('%s -- %s%s- %s Nexteer',NxtrConf,char(169),first,last)
      | end
  NVM Shadow RAM : DataStoreWrite  RequirementInfo={} %GIDa_1659f01a_6b97_4ff1_afb0_e4ba99927e44  DataStoreName=HwTq0OffsTrim
  NVM1 Shadow RAM : DataStoreWrite  RequirementInfo={'linktype_rmi_doors' '0000c468 (/ESG Group/FDD Module Requirements/EA4 Specific/CM650A_HwTq0Meas)' '#CM650A_49' 'true' 'REQ: CM650A_49' '' } %GIDa_340e34c7_c59a_43cb_a8d9_5aafb58ec96b  DataStoreName=HwTq0OffsTrimPrfmdSts
  Set : Constant
  Set Ram Block Status : NxtrNvM/Set Ram Block Status  FuncName=Set Ram Block Status  NvMBlockName=HwTq0Offs  VoidFuncRtn=on  BlockChanged_DSN=NvMSRBS_BlockChanged  Return_DSN=NvMSRBS_Return
      settings: AttributesFormatString=%<FuncName>
  Set3 : Constant  OutDataTypeStr=uint8
  wires:
  Set/1 -> NVM1 Shadow RAM/1
  HwTqWrTrimData/1 -> NVM Shadow RAM/1
  Set3/1 -> Set Ram Block Status/1

== system CM650A_HwTq0Meas/HwTq0Meas/HwTq0MeasInit1 ==
  note: Follow below steps in same order:
      |
      | 1. Enable Configuration mode, RSENT0MDC.OMC = 1U
      | 2. Verify whether peripheral is in Configuration mode RSENT0MST.OMS ==1U and wait till 2us* ,it is in configuration mode
      | 3. Configure the SENT Register as per  "CM650A_HwTq0Meas_RSENTPeripheralCfg.xlsx"
      | 4. Enable Operation active mode, RSENT0MDC.OMC = 5U
      | 5. Verify whether peripheral is in Opertation active mode RSENT0MST.OMS ==5U and wait till 2us* ,it is in Opertation active mode
      | 6. Client Call "IoHwAb_SetFctPrphlHwTq0"- Port Configuration shall change to output in alternate mode from default input for RSENT0 SPCO IO pin.
      |
      | Note: * - actual minimum is 150ns as per Scott Winder email from Renesas
  function : TriggerPort  TriggerType=falling
  CopyRight2 : Subsystem  Description=|  mask(Copyright Information){none=on}
      | Copyright info block.                                               
      |                                                                     
      | Place copyright information at the top of every subsystem in design.
      mask prompts: none "No parameters"
      mask help: Place copyright information at the top of every subsystem in design.
      mask Display:
      | NxtrConf = 'Nexteer Confidential';
      | 
      | sys = bdroot; %handle for the current model ("system")
      | first = get_param(sys,'Created');
      | first = first(end-3:end);  %year is last four digits
      | 
      | last = get_param(sys,'LastModifiedDate');
      | if isempty(last)
      |     last = datestr(now,'yyyy');
      | else
      |     last = last(end-3:end);
      | end
      | 
      | if strcmp(first,last)
      |     fprintf('%s -- Copyright %s Nexteer',NxtrConf,first)
      | else
      |     fprintf('%s -- %s%s- %s Nexteer',NxtrConf,char(169),first,last)
      | end
  GetRefTmr1MicroSec32bit : Subsystem
      settings: AttributesFormatString=Client Call : Start Time
  GetTiSpan1MicroSec32bit : Subsystem
  IoHwAb_SetFctPrphlHwTq0 : Subsystem
  Terminator1 : Terminator
  wires:
  GetRefTmr1MicroSec32bit/1(RefTmr) -> GetTiSpan1MicroSec32bit/1(RefTmr)
  GetTiSpan1MicroSec32bit/1(TiSpan) -> Terminator1/1

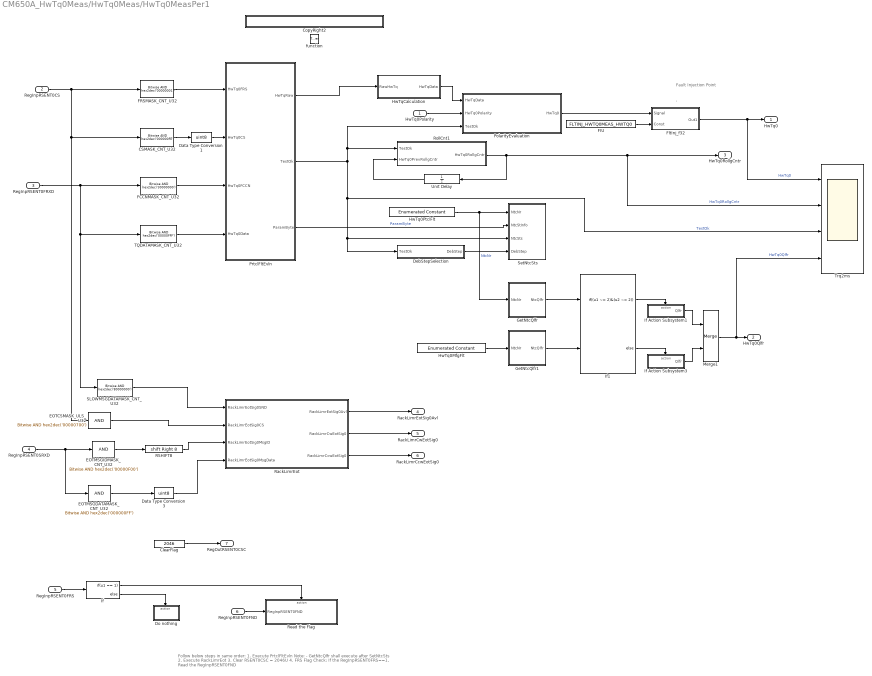
== system CM650A_HwTq0Meas/HwTq0Meas/HwTq0MeasPer1 ==
  note: ,
  note: Fault
      | Injection
      | Point
  note: Follow below steps in same order:
      |
      | 1. Execute PrtclFltEvln
      | Note: - GetNtcQlfr shall execute after SetNtcSts
      | 2. Execute RackLimrEot
      | 3. Clear RSENT0CSC = 2046U
      | 4. FRS Flag Check: If the RegInpRSENT0FRS==1,  Read the RegInpRSENT0FND
  HwTq0Polarity : Inport
  RegInpRSENT0CS : Inport  Port=2
  RegInpRSENT0FRXD : Inport  Port=3
  RegInpRSENT0SRXD : Inport  Port=4
  RegInpRSENT0FRS : Inport  Port=5
  RegInpRSENT0FND : Inport  Port=6
  function : TriggerPort  TriggerType=function-call
  CSMASK_CNT_U32 : simulink/Logic and Bit Operations/Bitwise Operator  logicop=AND  UseBitMask=on  BitMask=hex2dec('000000FE')  BitMaskRealWorld=Stored Integer
  ClearFlag : Constant  RequirementInfo={} %GIDa_7eee2515_59c0_4ccf_8b91_a4e4e3d831bb  Value=2046  OutDataTypeStr=uint16
  CopyRight2 : Subsystem  Description=|  mask(Copyright Information){none=on}
      | Copyright info block.                                               
      |                                                                     
      | Place copyright information at the top of every subsystem in design.
      mask prompts: none "No parameters"
      mask help: Place copyright information at the top of every subsystem in design.
      mask Display:
      | NxtrConf = 'Nexteer Confidential';
      | 
      | sys = bdroot; %handle for the current model ("system")
      | first = get_param(sys,'Created');
      | first = first(end-3:end);  %year is last four digits
      | 
      | last = get_param(sys,'LastModifiedDate');
      | if isempty(last)
      |     last = datestr(now,'yyyy');
      | else
      |     last = last(end-3:end);
      | end
      | 
      | if strcmp(first,last)
      |     fprintf('%s -- Copyright %s Nexteer',NxtrConf,first)
      | else
      |     fprintf('%s -- %s%s- %s Nexteer',NxtrConf,char(169),first,last)
      | end
  Data Type Conversion1 : DataTypeConversion  OutDataTypeStr=uint8
  Data Type Conversion3 : DataTypeConversion  OutDataTypeStr=uint8
  DebStepSelection : Subsystem
  Do nothing : Subsystem  RequirementInfo={} %GIDa_4f5e3310_e958_4ca7_9a68_f10a8a1034f5  TreatAsAtomicUnit=on
  EOTCSMASK_ULS_U32 : simulink/Logic and Bit Operations/Bitwise Operator  logicop=AND  UseBitMask=on  BitMask=hex2dec('00000700')  BitMaskRealWorld=Stored Integer
  EOTMSGDATAMASK_CNT_U32 : simulink/Logic and Bit Operations/Bitwise Operator  logicop=AND  UseBitMask=on  BitMask=hex2dec('000000FF')  BitMaskRealWorld=Stored Integer
  EOTMSGIDMASK_CNT_U32 : simulink/Logic and Bit Operations/Bitwise Operator  logicop=AND  UseBitMask=on  BitMask=hex2dec('00000F00')  BitMaskRealWorld=Stored Integer
  FCCNMASK_CNT_U32 : simulink/Logic and Bit Operations/Bitwise Operator  logicop=AND  UseBitMask=on  BitMask=hex2dec('30000000')  BitMaskRealWorld=Stored Integer
  FIU : Constant  Value=FLTINJ_HWTQ0MEAS_HWTQ0
  FRSMASK_CNT_U32 : simulink/Logic and Bit Operations/Bitwise Operator  logicop=AND  UseBitMask=on  BitMask=hex2dec('00000001')  BitMaskRealWorld=Stored Integer
  FltInj_f32 : Subsystem  RequirementInfo={'linktype_rmi_doors' '0000c468 (/ESG Group/FDD Module Requirements/EA4 Specific/CM650A_HwTq0Meas)' '#CM650A_57' 'true' 'REQ: CM650A_57' '' } %GIDa_2fc4bfb2_aa92_4a62_a009_934dcc687090  TreatAsAtomicUnit=on  VariantControl=FltInj_sim  mask(Fault_Injection){}
      mask help: Fault Injection is a simulation only block for EA4 programs.
  GetNtcQlfr : Subsystem
  GetNtcQlfr1 : Subsystem
  HwTq0MfgFlt : simulink/Sources/Enumerated Constant  OutDataTypeStr=Enum: NtcNr1  Value=NtcNr1.NTCNR_0X1E0  SampleTime=inf
  HwTq0PtclFlt : simulink/Sources/Enumerated Constant  OutDataTypeStr=Enum: NtcNr1  Value=NtcNr1.NTCNR_0X073  SampleTime=inf
  HwTqCalculation : Subsystem
  If : If  RequirementInfo={} %GIDa_1f4eae7f_3e40_4d46_9f43_a9ba329a02a3  IfExpression=u1 == 1
  If Action Subsystem1 : Subsystem  TreatAsAtomicUnit=on
  If Action Subsystem3 : Subsystem  TreatAsAtomicUnit=on
  If1 : If  NumInputs=2  IfExpression=(u1 ~= 2)&(u2 ~= 2)
  Merge1 : Merge
  PolarityEvaluation : Subsystem  RequirementInfo={'linktype_rmi_doors' '0000c468 (/ESG Group/FDD Module Requirements/EA4 Specific/CM650A_HwTq0Meas)' '#CM650A_24' 'true' 'REQ: CM650A_24' '' ; 'linktype_rmi_doors' '0000c468 (/ESG Group/FDD Module Requirements/EA4 Specific/CM650A_HwTq0Meas)' '#CM650A_27' 'true' 'REQ: CM650A_27' '' } %GIDa_7dd0f124_da9d_41af_bfd5_c8f0b8205e28
  PrtclFltEvln : Subsystem
  RSHIFT8 : ArithShift  BitShiftNumber=8  BitShiftDirection=Right
  RackLimrEot : Subsystem
  Read the Flag : Subsystem  RequirementInfo={} %GIDa_acf6a32f_9290_45d4_a622_d96164b6a9fb  TreatAsAtomicUnit=on
  RollCnt1 : Stateflow chart  RequirementInfo={} %GIDa_be1c412e_1791_4e7e_9b3e_cc09ba9a6629  TreatAsAtomicUnit=on
  SLOWMSGDATAMASK_CNT_U32 : simulink/Logic and Bit Operations/Bitwise Operator  logicop=AND  UseBitMask=on  BitMask=hex2dec('80000000')  BitMaskRealWorld=Stored Integer
  SetNtcSts : Subsystem  RequirementInfo={'linktype_rmi_doors' '0000c468 (/ESG Group/FDD Module Requirements/EA4 Specific/CM650A_HwTq0Meas)' '#CM650A_34' 'true' 'REQ: CM650A_34' '' } %GIDa_7c28da3a_b49c_4a2c_9776_430afb4b2413
  TQDATAMASK_CNT_U32 : simulink/Logic and Bit Operations/Bitwise Operator  logicop=AND  UseBitMask=on  BitMask=hex2dec('00000FFF')  BitMaskRealWorld=Stored Integer
  Trq2ms : Scope  NumInputPorts=4
      settings: YMin=-10~0~1.9~1  YMax=10~275~2.1~2  SaveName=ScopeData3
  Unit Delay : UnitDelay  SampleTime=-1  StateName=HwTq0MeasPrevRollgCntr  StateMustResolveToSignalObject=on
      settings: AttributesFormatString=%<StateName>
  HwTq0 : Outport  RequirementInfo={} %GIDa_3b2abd0f_dff5_44f3_b788_adb2172836f5
  HwTq0Qlfr : Outport  RequirementInfo={'linktype_rmi_doors' '0000c468 (/ESG Group/FDD Module Requirements/EA4 Specific/CM650A_HwTq0Meas)' '#CM650A_25' 'true' 'REQ: CM650A_25' '' } %GIDa_5eff5979_1038_44df_a727_ac7fcfb158b0  Port=2
  HwTq0RollgCntr : Outport  RequirementInfo={'linktype_rmi_doors' '0000c468 (/ESG Group/FDD Module Requirements/EA4 Specific/CM650A_HwTq0Meas)' '#CM650A_26' 'true' 'REQ: CM650A_26' '' } %GIDa_de83414f_64c7_40b0_8047_6b8baba686d2  Port=3
  RackLimrEotSig0Avl : Outport  RequirementInfo={} %GIDa_5152d964_4fd2_4e97_b84e_a43b7a360335  Port=4
  RackLimrCwEotSig0 : Outport  RequirementInfo={} %GIDa_01cac5ef_4b3d_4695_98b7_d096beea4adb  Port=5
  RackLimrCcwEotSig0 : Outport  RequirementInfo={} %GIDa_46f09250_9d89_47f9_9dfb_d1a8f900c9d1  Port=6
  RegOutRSENT0CSC : Outport  Port=7
  wires:
  PrtclFltEvln/1(HwTqRaw) -> HwTqCalculation/1(RawHwTq)
  HwTqCalculation/1(HwTqData) -> PolarityEvaluation/1(HwTqData)
  PrtclFltEvln/2(TestOk) -> PolarityEvaluation/3(TestOk), RollCnt1/1(TestOk), Trq2ms/3, SetNtcSts/3(NtcSts), DebStepSelection/1(TestOk)  "TestOk"
  HwTq0Polarity/1 -> PolarityEvaluation/2(HwTq0Polarity)
  HwTq0PtclFlt/1 -> GetNtcQlfr/1(NtcNr), SetNtcSts/1(NtcNr)  "NtcNr"
  PrtclFltEvln/3(ParamByte) -> SetNtcSts/2(NtcStInfo)  "ParamByte"
  DebStepSelection/1(DebStep) -> SetNtcSts/4(DebStep)
  FltInj_f32/1(Out1) -> HwTq0/1, Trq2ms/1  "HwTq0"
  RollCnt1/1(HwTq0RollgCntr) -> Trq2ms/2, HwTq0RollgCntr/1, Unit Delay/1  "HwTq0RollgCntr"
  Unit Delay/1 -> RollCnt1/2(HwTq0PrevRollgCntr)
  FIU/1 -> FltInj_f32/2(Const)
  PolarityEvaluation/1(HwTq0) -> FltInj_f32/1(Signal)
  HwTq0MfgFlt/1 -> GetNtcQlfr1/1(NtcNr)
  GetNtcQlfr/1(NtcQlfr) -> If1/1
  GetNtcQlfr1/1(NtcQlfr) -> If1/2
  If Action Subsystem1/1(Qlfr) -> Merge1/1
  If Action Subsystem3/1(Qlfr) -> Merge1/2
  Merge1/1 -> Trq2ms/4, HwTq0Qlfr/1  "HwTq0Qlfr"
  If1/2 -> If Action Subsystem3/Action
  If1/1 -> If Action Subsystem1/Action
  RegInpRSENT0FRXD/1 -> TQDATAMASK_CNT_U32/1, SLOWMSGDATAMASK_CNT_U32/1, FCCNMASK_CNT_U32/1
  RegInpRSENT0CS/1 -> CSMASK_CNT_U32/1, EOTCSMASK_ULS_U32/1, FRSMASK_CNT_U32/1
  RackLimrEot/1(RackLimrEotSig0Avl) -> RackLimrEotSig0Avl/1
  RackLimrEot/2(RackLimrCwEotSig0) -> RackLimrCwEotSig0/1
  RackLimrEot/3(RackLimrCcwEotSig0) -> RackLimrCcwEotSig0/1
  CSMASK_CNT_U32/1 -> Data Type Conversion1/1
  TQDATAMASK_CNT_U32/1 -> PrtclFltEvln/4(HwTq0Data)
  FCCNMASK_CNT_U32/1 -> PrtclFltEvln/3(HwTq0FCCN)
  FRSMASK_CNT_U32/1 -> PrtclFltEvln/1(HwTq0FRS)
  EOTCSMASK_ULS_U32/1 -> RackLimrEot/2(RackLimrEotSig0CS)
  SLOWMSGDATAMASK_CNT_U32/1 -> RackLimrEot/1(RackLimrEotSig0SND)
  RegInpRSENT0SRXD/1 -> EOTMSGDATAMASK_CNT_U32/1, EOTMSGIDMASK_CNT_U32/1
  EOTMSGIDMASK_CNT_U32/1 -> RSHIFT8/1
  EOTMSGDATAMASK_CNT_U32/1 -> Data Type Conversion3/1
  RSHIFT8/1 -> RackLimrEot/3(RackLimrEotSig0MsgID)
  Data Type Conversion1/1 -> PrtclFltEvln/2(HwTq0CS)
  Data Type Conversion3/1 -> RackLimrEot/4(RackLimrEotSig0MsgData)
  ClearFlag/1 -> RegOutRSENT0CSC/1
  RegInpRSENT0FRS/1 -> If/1
  If/1 -> Read the Flag/Action
  If/2 -> Do nothing/Action
  RegInpRSENT0FND/1 -> Read the Flag/1(RegInpRSENT0FND)

== system CM650A_HwTq0Meas/HwTq0Meas/HwTq0MeasPer2 ==
  note: Information Only:
      | - Trim not performed Ntc
  function : TriggerPort  TriggerType=function-call
  CopyRight2 : Subsystem  Description=|  mask(Copyright Information){none=on}
      | Copyright info block.                                               
      |                                                                     
      | Place copyright information at the top of every subsystem in design.
      mask prompts: none "No parameters"
      mask help: Place copyright information at the top of every subsystem in design.
      mask Display:
      | NxtrConf = 'Nexteer Confidential';
      | 
      | sys = bdroot; %handle for the current model ("system")
      | first = get_param(sys,'Created');
      | first = first(end-3:end);  %year is last four digits
      | 
      | last = get_param(sys,'LastModifiedDate');
      | if isempty(last)
      |     last = datestr(now,'yyyy');
      | else
      |     last = last(end-3:end);
      | end
      | 
      | if strcmp(first,last)
      |     fprintf('%s -- Copyright %s Nexteer',NxtrConf,first)
      | else
      |     fprintf('%s -- %s%s- %s Nexteer',NxtrConf,char(169),first,last)
      | end
  Data Store Read1 : DataStoreRead  DataStoreName=HwTq0OffsTrimPrfmdSts
  Ground : Ground
  HwTq0MfgFlt : simulink/Sources/Enumerated Constant  OutDataTypeStr=Enum: NtcNr1  Value=NtcNr1.NTCNR_0X1E0  SampleTime=inf
  If : If  IfExpression=(u1 ~= 0)
  If Action Subsystem : Subsystem  RequirementInfo={'linktype_rmi_doors' '0000c468 (/ESG Group/FDD Module Requirements/EA4 Specific/CM650A_HwTq0Meas)' '#CM650A_67' 'true' 'REQ: CM650A_67' '' } %GIDa_eda0e9fe_0ef4_4d37_918c_815346a1604f  TreatAsAtomicUnit=on
  If Action Subsystem1 : Subsystem  RequirementInfo={'linktype_rmi_doors' '0000c468 (/ESG Group/FDD Module Requirements/EA4 Specific/CM650A_HwTq0Meas)' '#CM650A_65' 'true' 'REQ: CM650A_65' '' } %GIDa_f1a05e9a_fff8_4eab_8b85_2e72f495a740  TreatAsAtomicUnit=on
  Merge : Merge
  Merge1 : Merge
  Scope : Scope  NumInputPorts=2
      settings: YMin=-5~-5  YMax=5~5  SaveName=ScopeData3
  SetNtcSts : Subsystem  RequirementInfo={'linktype_rmi_doors' '0000c468 (/ESG Group/FDD Module Requirements/EA4 Specific/CM650A_HwTq0Meas)' '#CM650A_61' 'true' 'REQ: CM650A_61' '' } %GIDa_03dde2fd_062f_4b23_859a_fc5579118954
  wires:
  Ground/1 -> SetNtcSts/4(DebStep)
  HwTq0MfgFlt/1 -> SetNtcSts/1(NtcNr)
  Data Store Read1/1 -> If/1
  If/1 -> If Action Subsystem/Action
  If/2 -> If Action Subsystem1/Action
  If Action Subsystem/1(ParamByte) -> Merge/1
  If Action Subsystem1/1(ParamByte) -> Merge/2
  If Action Subsystem/2(TestOk) -> Merge1/1
  If Action Subsystem1/2(TestOk) -> Merge1/2
  Merge/1 -> Scope/1, SetNtcSts/2(NtcStInfo)  "ParamByte"
  Merge1/1 -> Scope/2, SetNtcSts/3(NtcSts)  "TestOk"
